simulink model "ssc_hydraulic_actuator_analog_control"  (R2020a)
settings: Solver=VariableStepAuto  StartTime=0.0  StopTime=10  MaxStep=0.02  RelTol=1e-3  AbsTol=1e-3  EnableMultiTasking=on
libraries: fl_lib x66, nesl_utility x3
CloseFcn:
  | try,close(h1_ssc_hydraulic_actuator_analog_control),end
  | clear h1_ssc_hydraulic_actuator_analog_control
  | 
  | clear simlog_ssc_hydraulic_actuator_analog_control
Description:
  | Hydraulic Actuator with Analog Position Controller
settings Model: Creator=MathWorks  LastModifiedBy=victo
settings SolverCC: AutoScaleAbsTol=off
settings DataIOCC: LimitDataPoints=on  SaveFormat=Array  ReturnWorkspaceOutputs=off
settings OptimizationCC: LifeSpan=inf
settings DebuggingCC: SolverPrmCheckMsg=warning  AllowSymbolicDim=off  PregeneratedLibrarySubsystemCodeDiagnostic=none  SFUnexpectedBacktrackingDiag=warning  SFNoUnconditionalDefaultTransitionDiag=warning  SFExecutionAtInitializationDiag=none  ArithmeticOperatorsInVariantConditions=warning
settings HardwareCC: ProdBitPerPointer=32  ProdBitPerSizeT=32  ProdBitPerPtrDiffT=32  ProdLargestAtomicFloat=None  ProdIntDivRoundTo=Undefined  ProdEndianess=Unspecified  ProdWordSize=32  ProdHWDeviceType=32-bit Generic
settings ModelReferenceCC: PropagateSignalLabelsOutOfModel=off
settings SFSimCC: SimUseLocalCustomCode=off  CustomCodeUndefinedFunction=UseInterfaceOnly
settings RTWCC: RTWUseLocalCustomCode=off
settings CodeAppCC: StateflowObjectComments=on
settings GRTTargetCC: TargetLangStandard=C89/C90 (ANSI)
settings ConfigComp: CovMetricSettings=dw  CovHtmlReporting=on  CovSaveCumulativeToWorkspaceVar=on  CovSaveSingleToWorkspaceVar=on  CovExternalEMLEnable=off  CovSFcnEnable=off
settings SimscapeCC: SimscapeLogType=all  SimscapeLogSimulationStatistics=on  SimscapeLogName=simlog_ssc_hydraulic_actuator_analog_control  SimscapeLogDataHistory=10000

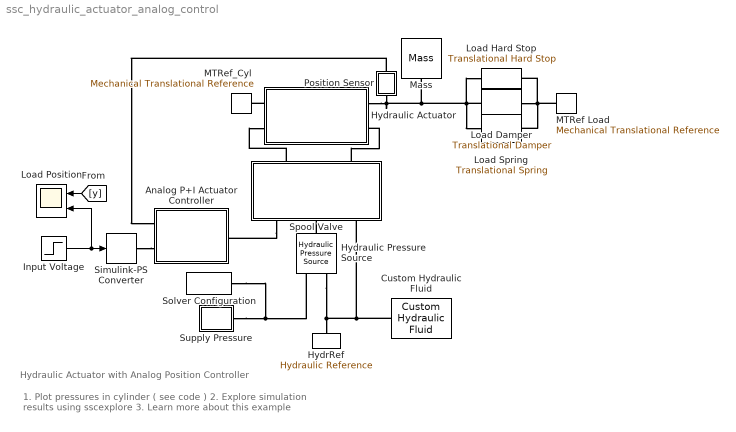
== system ssc_hydraulic_actuator_analog_control ==
  note: 1. Plot pressures in cylinder ( see code )
      | 2. Explore simulation results using sscexplore
      | 3. Learn more about this example
  note: Hydraulic Actuator with Analog Position Controller
  Analog P+I Actuator Controller : Subsystem
  Custom Hydraulic Fluid : fl_lib/Hydraulic/Hydraulic Utilities/Custom Hydraulic Fluid  density=850 kg/m^3  viscosity_kin=1.8e-05 m^2/s  bulk=8e+08 Pa  alpha=0.005  range_error=2
      settings: SourceProductName=Foundation Library  InternalSimscapePortConfiguration="{\"Bottom\":[],\"Left\":[],\"Right\":[{\"id\":\"G\",\"label\":\"\",\"type\":\"foundation.hydraulic.hydraulic\"}],\"Top\":[]}"
  HydrRef : fl_lib/Hydraulic/Hydraulic Elements/Hydraulic Reference
      settings: SourceProductName=Foundation Library
  Hydraulic Pressure Source : fl_lib/Hydraulic/Hydraulic Sources/Hydraulic Pressure Source
      settings: SourceProductName=Foundation Library  InternalSimscapePortConfiguration="{\"Bottom\":[],\"Left\":[{\"id\":\"P\",\"label\":\"P\",\"type\":\"foundation.hydraulic.hydraulic\"}],\"Right\":[{\"id\":\"S\",\"label\":\"S\",\"type\":\"input\"},{\"id\":\"T\",\"label\":\"T\",\"type\":\"foundation.hydraulic.hydraulic\"}],\"Top\":[]}"
  Hydraulic Actuator : Subsystem  mask(Double-Acting Hydraulic Actuator){A=5e-4, V=10e-6, PA=100, PB=100}
      mask prompts: A "Piston area (m^2)"; V "Chamber dead volume (m^3)"; PA "Positive-acting chamber A initial pressure (bar)"; PB "Negative-acting chamber B initial pressure (bar)"
      mask help: Models a double-acting hydraulic actuator using foundation library blocks
      mask Display:
      | plot([127.790967235342;156.136468285695;156.136468285695;127.790967235342;127.790967235342], [113.618216710165;113.618216710165;56.927214609459;56.927214609459;113.618216710165])
      | plot([261.014822172001;326.209474587813], [85.2727156598121;85.2727156598121])
      | plot([212.827470386401;212.827470386401;326.209474587813], [56.927214609459;28.581713559106;28.581713559106])
      | patch([0;326.445687096566;326.445687096566;0;0;0.472425017505884;0.472425017505884;325.97326207906;325.97326207906;0.472425017505884;0], [113.854429218918;113.854429218918;0;0;113.854429218918;113.382004201412;0.472425017505884;0.472425017505884;113.382004201412;113.382004201412;113.854429218918], [1;1;1])
      | plot([227.000220911577;227.000220911577;82.4381655547768;82.4381655547768;227.000220911577;227.000220911577], [99.4454661849886;113.618216710165;113.618216710165;56.927214609459;56.927214609459;71.0999651346356])
      | plot([82.4381655547768;54.0926645044237;82.4381655547768], [113.618216710165;85.2727156598121;56.927214609459])
      | plot([156.136468285695;261.014822172001;261.014822172001;156.136468285695;156.136468285695], [99.4454661849886;99.4454661849886;71.0999651346356;71.0999651346356;99.4454661849886])
      | plot([0.236212508752942;110.78366660513;110.78366660513], [28.581713559106;28.581713559106;56.927214609459])
      | plot([54.0926645044237;0.236212508752942], [85.2727156598121;85.2727156598121])
      | 
      | color('red');
      | port_label('LConn',1,'C');
      | port_label('LConn',2,'A');
      | port_label('RConn',1,'R');
      | port_label('RConn',2,'B');
      | color('black');
  Input Voltage : Step  Time=0.2  Before=2.5  After=3.0  SampleTime=0
  Load Position : Scope  NumInputPorts=2
  Load Damper : fl_lib/Mechanical/Translational Elements/Translational Damper  D=5000 N/(m/s)  v_specify=off  v_priority=High  v=0 m/s  v_nominal_specify=off  v_nominal_unit=m/s  v_nominal_value=1  f_specify=off  f_priority=High  f=0 N  f_nominal_specify=off  f_nominal_unit=N  f_nominal_value=1
      settings: SourceProductName=Foundation Library
  Load Hard Stop : fl_lib/Mechanical/Translational Elements/Translational Hard Stop  upper_bnd=50 mm  lower_bnd=-50 mm  stiff_up=1e+07 N/m  stiff_low=1e+07 N/m  D_up=3000 N/(m/s)  D_low=3000 N/(m/s)  model=3  transition=0.1 mm  v_specify=off  v_priority=High  v=0 m/s  v_nominal_specify=off  v_nominal_unit=m/s  v_nominal_value=1  f_specify=off  f_priority=High  f=0 N  f_nominal_specify=off  f_nominal_unit=N  f_nominal_value=1  x_specify=on  x_priority=High  x=0 m  x_nominal_specify=off  x_nominal_unit=m  x_nominal_value=1
      settings: SourceProductName=Foundation Library
  Load Spring : fl_lib/Mechanical/Translational Elements/Translational Spring  spr_rate=100000 N/m  v_specify=off  v_priority=High  v=0 m/s  v_nominal_specify=off  v_nominal_unit=m/s  v_nominal_value=1  f_specify=off  f_priority=High  f=0 N  f_nominal_specify=off  f_nominal_unit=N  f_nominal_value=1  x_specify=off  x_priority=High  x=0 mm  x_nominal_specify=off  x_nominal_unit=m  x_nominal_value=1
      settings: SourceProductName=Foundation Library
  MTRef Load : fl_lib/Mechanical/Translational Elements/Mechanical Translational Reference
      settings: SourceProductName=Foundation Library
  MTRef_Cyl : fl_lib/Mechanical/Translational Elements/Mechanical Translational Reference
      settings: SourceProductName=Foundation Library
  Mass : fl_lib/Mechanical/Translational Elements/Mass  mass=20 kg  v_specify=off  v_priority=High  v=0 m/s  v_nominal_specify=off  v_nominal_unit=m/s  v_nominal_value=1  f_specify=off  f_priority=High  f=0 N  f_nominal_specify=off  f_nominal_unit=N  f_nominal_value=1
      settings: SourceProductName=Foundation Library
  Position Sensor : Subsystem
      mask Display: disp('y')
  Simulink-PS Converter : nesl_utility/Simulink-PS Converter  PhysicalDomain=network_engine_domain  SubClassName=ps_input  LeftPortType=input  RightPortType=output  PseudoPeriodic=off  Frequencies=[]  NoiseDistribution=none  NoiseParameters=[]  Unit=V  AffineConversion=off  FilteringAndDerivatives=zero  SimscapeFilterOrder=1  InputFilterTimeConstant=.001  UdotUserProvided=0
      settings: SourceProductName=Utilities
  Solver Configuration : nesl_utility/Solver Configuration  PhysicalDomain=network_engine_domain  SubClassName=solver  LeftPortType=input  RightPortType=generic  Tones=[]  Harmonics=[]  SimulateNoise=off  Profile=off  UseLocalSampling=off  EnableSwitchedLinearOptims=on  FrequencyDomain=off  UseCCode=off  RelTol=0.001  AbsTol=1e-06  MinStep=1e-09  ToWorkspace=off  RevertToSquareIcSolve=off  NumHomotopyIterations=100  PhasorMode=off  PhasorModeNumHarmonics=1  DoDC=off  ResidualTolerance=1e-9  UseLocalSolver=off  LocalSolverChoice=NE_BACKWARD_EULER_ADVANCER  LocalSolverSampleTime=0.001  DoFixedCost=off  MaxNonlinIter=3  MaxModeIter=2  LinearAlgebra=auto  EquationFormulation=NE_TIME_EF  DelaysMemoryBudget=1024  AutomaticFiltering=on  FilteringTimeConstant=0.001  PartitionStorageMethod=AS_NEEDED  PartitionMemoryBudget=1024  PartitionMethod=ROBUST
      settings: SourceProductName=Utilities
  Spool Valve : Subsystem  Tag=PublishSubsystem  mask(Single-Stage Servo Valve){K_V=0.5, x_max=0.5, A_max=9, x_lap=0.02, A_leak=0.25, G=0.5e-3/(pi/2), J=1e-4, lambda=0.01, R=10, L=2.5, Kt=0.04, R_controller=[10e3 10e3 10e3 100e3 50 100e3 10e3]}
      mask prompts: K_V "Flow Coefficient:"; x_max "Spool displacement limit (mm)"; A_max "Maximum orifice area (mm^2)"; x_lap "Spool displacement range for leakage (mm)"; A_leak "Leakage area at x=0 (mm^2)"; G "Spool displacement per motor rotation (m/radian)"; J "Total inertia reflected to motor (kg m^2)"; lambda "Total damping reflected to motor (Nm/(rad/s))"; R "Torque motor winding resistance (ohms)"; L "Torque motor winding inductance (H)"; Kt "Torque motor torque constant (Nm/A)"; R_controller "Motor controller resistance values [R1 R2 R3 R4 R5 R6 R7] (ohms)"
      mask help: Models a spool valve actuated directly by a torque motor.
      mask Display:
      | % Plot icon
      | plot([0;337.311462499201;337.311462499201;0;0], [566.910021007061;566.910021007061;0;0;566.910021007061])
      | plot([84.6585631370544;241.503668949008], [353;353])
      | plot([84.6585631370544;241.503668949008], [214;214])
      | plot([84.6585631370544;241.503668949008;241.503668949008;84.6585631370544;84.6585631370544], [491;491;76;76;491])
      | plot([84.6585631370544;241.503668949008], [449;449])
      | plot([241.503668949008;210.071657784283], [310;310])
      | plot([210.071657784283;210.071657784283;210.071657784283], [326;295;310.414731502533])
      | plot([241.503668949008;210.071657784283], [257;257])
      | plot([210.071657784283;210.071657784283;210.071657784283], [272;241;236.464468762279])
      | plot([84.6585631370544;115.964594297111], [257;257])
      | plot([115.964594297111;115.964594297111;115.964594297111], [272;241;236.464468762279])
      | plot([84.6585631370544;115.964594297111], [310;310])
      | plot([115.964594297111;115.964594297111;115.964594297111], [326;295;310.414731502533])
      | plot([84.6585631370544;241.503668949008], [185;110])
      | plot([241.503668949008;84.6585631370544], [185;110])
      | plot([84.6585631370544;241.503668949008], [395;395])
      | patch([85.0365031510592;110.547454096377;121.885654516518;85.0365031510592], [110;140;120;110], [0;0;0])
      | plot([85.0365031510592;110.547454096377;121.885654516518;85.0365031510592], [110;140;120;110])
      | patch([240.936758928001;204.087607562542;215.425807982683;240.936758928001], [109;120;140;109], [0;0;0])
      | 
      | plot([240.936758928001;204.087607562542;215.425807982683;240.936758928001], [109;120;140;109])
      | patch([83.6507230997086;127.554754726589;127.554754726589;83.6507230997086], [394;405;384;394], [0;0;0])
      | plot([83.6507230997086;127.554754726589;127.554754726589;83.6507230997086], [394;405;384;394])
      | patch([245.283069089055;201.253057457507;201.253057457507;245.283069089055], [451;461;440;451], [0;0;0])
      | plot([245.283069089055;201.253057457507;201.253057457507;245.283069089055], [451;461;440;451])
      | 
      | % Port labels
      | color('red')
      | port_label('LConn', 1,'S')
      | port_label('LConn', 2,'P')
      | port_label('LConn', 3,'T')
      | port_label('RConn', 1,'A')
      | port_label('RConn', 2,'B')
      | color('black')
  Supply Pressure : Subsystem
  wires:
  Input Voltage/1 -> Load Position/2, Simulink-PS Converter/1
  [y] -> Load Position/1
  connections:
  Spool Valve/LConn1 -- Analog P+I Actuator Controller/RConn1
  Custom Hydraulic Fluid/RConn1 -- Hydraulic Pressure Source/RConn2 -- HydrRef/LConn1 -- Spool Valve/LConn3
  Spool Valve/RConn2 -- Hydraulic Actuator/RConn2
  Spool Valve/RConn1 -- Hydraulic Actuator/LConn2
  Simulink-PS Converter/RConn1 -- Analog P+I Actuator Controller/LConn2
  Hydraulic Pressure Source/LConn1 -- Spool Valve/LConn2
  Load Spring/LConn1 -- Load Damper/LConn1 -- Mass/LConn1 -- Position Sensor/RConn1 -- Hydraulic Actuator/RConn1 -- Load Hard Stop/LConn1
  Position Sensor/LConn1 -- Analog P+I Actuator Controller/LConn1
  Hydraulic Actuator/LConn1 -- MTRef_Cyl/LConn1
  Supply Pressure/RConn1 -- Solver Configuration/RConn1 -- Hydraulic Pressure Source/RConn1
  Load Hard Stop/RConn1 -- Load Damper/RConn1 -- MTRef Load/LConn1 -- Load Spring/RConn1

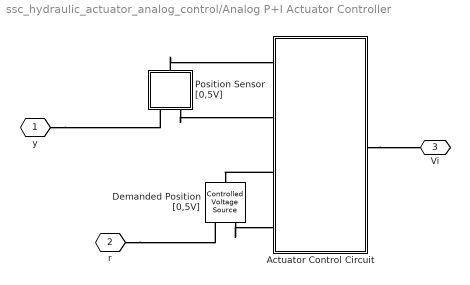
== system ssc_hydraulic_actuator_analog_control/Analog P+I Actuator Controller ==
  Actuator Control Circuit : Subsystem  Tag=PublishSubsystem
  Demanded Position [0,5V] : fl_lib/Electrical/Electrical Sources/Controlled Voltage Source
      settings: SourceProductName=Foundation Library
  Position Sensor [0,5V] : Subsystem
  y : PMIOPort  Tag=PMCPort  Side=Left
  r : PMIOPort  Tag=PMCPort  Port=2  Side=Left
  Vi : PMIOPort  Port=3  Side=Right
  connections:
  y/RConn1 -- Position Sensor [0,5V]/LConn1
  r/RConn1 -- Demanded Position [0,5V]/RConn1
  Actuator Control Circuit/LConn3 -- Demanded Position [0,5V]/LConn1
  Position Sensor [0,5V]/RConn1 -- Actuator Control Circuit/LConn1
  Position Sensor [0,5V]/LConn2 -- Actuator Control Circuit/LConn2
  Actuator Control Circuit/RConn1 -- Vi/RConn1
  Demanded Position [0,5V]/RConn2 -- Actuator Control Circuit/LConn4

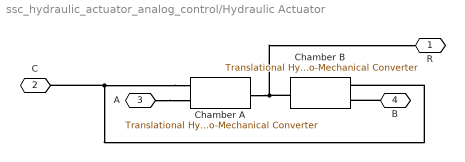
== system ssc_hydraulic_actuator_analog_control/Hydraulic Actuator ==
  Chamber A : fl_lib/Hydraulic/Hydraulic Elements/Translational Hydro-Mechanical Converter  area=A m^2  or=1  compressibility=1  init_pos=0 m  V_dead=V m^3  k_sh=1.4  initial_pressure=PA bar
      settings: SourceProductName=Foundation Library  InternalSimscapePortConfiguration="{\"Bottom\":[],\"Left\":[{\"id\":\"C\",\"label\":\"C\",\"type\":\"foundation.mechanical.translational.translational\"},{\"id\":\"A\",\"label\":\"A\",\"type\":\"foundation.hydraulic.hydraulic\"}],\"Right\":[{\"id\":\"R\",\"label\":\"R\",\"type\":\"foundation.mechanical.translational.translational\"}],\"Top\":[]}"
  Chamber B : fl_lib/Hydraulic/Hydraulic Elements/Translational Hydro-Mechanical Converter  area=A m^2  or=2  compressibility=1  init_pos=50 mm  V_dead=V m^3  k_sh=1.4  initial_pressure=PB bar
      settings: SourceProductName=Foundation Library  InternalSimscapePortConfiguration="{\"Bottom\":[],\"Left\":[{\"id\":\"C\",\"label\":\"C\",\"type\":\"foundation.mechanical.translational.translational\"},{\"id\":\"A\",\"label\":\"A\",\"type\":\"foundation.hydraulic.hydraulic\"}],\"Right\":[{\"id\":\"R\",\"label\":\"R\",\"type\":\"foundation.mechanical.translational.translational\"}],\"Top\":[]}"
  R : PMIOPort  Side=Right
  C : PMIOPort  Port=2  Side=Left
  A : PMIOPort  Port=3  Side=Left
  B : PMIOPort  Port=4  Side=Right
  connections:
  B/RConn1 -- Chamber B/LConn2
  Chamber A/RConn1 -- Chamber B/RConn1 -- R/RConn1
  A/RConn1 -- Chamber A/LConn2
  Chamber A/LConn1 -- C/RConn1 -- Chamber B/LConn1

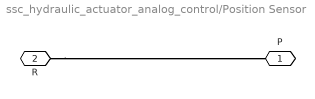
== system ssc_hydraulic_actuator_analog_control/Position Sensor ==
  P : PMIOPort  Side=Left
  R : PMIOPort  Port=2  Side=Right
  connections:
  R/RConn1 -- P/RConn1

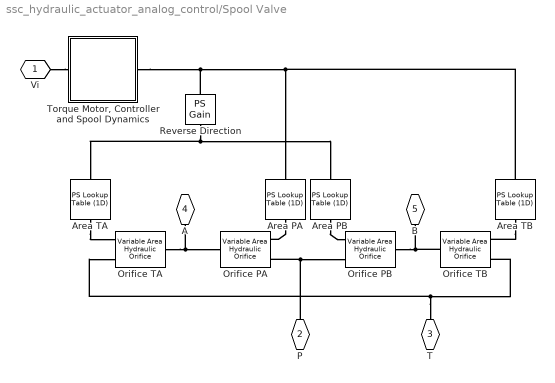
== system ssc_hydraulic_actuator_analog_control/Spool Valve ==
  Area PA : fl_lib/Physical Signals/Lookup Tables/PS Lookup Table (1D)  x=[-x_max -x_lap 0 x_lap x_max 2*x_max] mm  f=[0 0 A_leak 2*A_leak A_max A_max] mm^2  interp_method=simscape.enum.interpolation.linear  extrap_method=simscape.enum.extrapolation.linear
      settings: SourceProductName=Foundation Library
  Area PB : fl_lib/Physical Signals/Lookup Tables/PS Lookup Table (1D)  x=[-x_max -x_lap 0 x_lap x_max 2*x_max] mm  f=[0 0 A_leak 2*A_leak A_max A_max] mm^2  interp_method=simscape.enum.interpolation.linear  extrap_method=simscape.enum.extrapolation.linear
      settings: SourceProductName=Foundation Library
  Area TA : fl_lib/Physical Signals/Lookup Tables/PS Lookup Table (1D)  x=[-x_max -x_lap 0 x_lap x_max 2*x_max] mm  f=[0 0 A_leak 2*A_leak A_max A_max] mm^2  interp_method=simscape.enum.interpolation.linear  extrap_method=simscape.enum.extrapolation.linear
      settings: SourceProductName=Foundation Library
  Area TB : fl_lib/Physical Signals/Lookup Tables/PS Lookup Table (1D)  x=[-x_max -x_lap 0 x_lap x_max 2*x_max] mm  f=[0 0 A_leak 2*A_leak A_max A_max] mm^2  interp_method=simscape.enum.interpolation.linear  extrap_method=simscape.enum.extrapolation.linear
      settings: SourceProductName=Foundation Library
  Orifice PA : fl_lib/Hydraulic/Hydraulic Elements/Variable Area Hydraulic Orifice  C_d=K_V  min_area=1e-12 m^2  lam_spec=1  B_lam=0.999  Re_cr=12  q_specify=off  q_priority=High  q=1 m^3/s  q_nominal_specify=off  q_nominal_unit=m^3/s  q_nominal_value=1  p_specify=off  p_priority=High  p=0 Pa  p_nominal_specify=off  p_nominal_unit=Pa  p_nominal_value=1
      settings: SourceProductName=Foundation Library  InternalSimscapePortConfiguration="{\"Bottom\":[],\"Left\":[{\"id\":\"AR\",\"label\":\"AR\",\"type\":\"input\"},{\"id\":\"A\",\"label\":\"A\",\"type\":\"foundation.hydraulic.hydraulic\"}],\"Right\":[{\"id\":\"B\",\"label\":\"B\",\"type\":\"foundation.hydraulic.hydraulic\"}],\"Top\":[]}"
  Orifice PB : fl_lib/Hydraulic/Hydraulic Elements/Variable Area Hydraulic Orifice  C_d=K_V  min_area=1e-12 m^2  lam_spec=1  B_lam=0.999  Re_cr=12  q_specify=off  q_priority=High  q=1 m^3/s  q_nominal_specify=off  q_nominal_unit=m^3/s  q_nominal_value=1  p_specify=off  p_priority=High  p=0 Pa  p_nominal_specify=off  p_nominal_unit=Pa  p_nominal_value=1
      settings: SourceProductName=Foundation Library  InternalSimscapePortConfiguration="{\"Bottom\":[],\"Left\":[{\"id\":\"AR\",\"label\":\"AR\",\"type\":\"input\"},{\"id\":\"A\",\"label\":\"A\",\"type\":\"foundation.hydraulic.hydraulic\"}],\"Right\":[{\"id\":\"B\",\"label\":\"B\",\"type\":\"foundation.hydraulic.hydraulic\"}],\"Top\":[]}"
  Orifice TA : fl_lib/Hydraulic/Hydraulic Elements/Variable Area Hydraulic Orifice  C_d=K_V  min_area=1e-12 m^2  lam_spec=1  B_lam=0.999  Re_cr=12  q_specify=off  q_priority=High  q=1 m^3/s  q_nominal_specify=off  q_nominal_unit=m^3/s  q_nominal_value=1  p_specify=off  p_priority=High  p=0 Pa  p_nominal_specify=off  p_nominal_unit=Pa  p_nominal_value=1
      settings: SourceProductName=Foundation Library  InternalSimscapePortConfiguration="{\"Bottom\":[],\"Left\":[{\"id\":\"AR\",\"label\":\"AR\",\"type\":\"input\"},{\"id\":\"A\",\"label\":\"A\",\"type\":\"foundation.hydraulic.hydraulic\"}],\"Right\":[{\"id\":\"B\",\"label\":\"B\",\"type\":\"foundation.hydraulic.hydraulic\"}],\"Top\":[]}"
  Orifice TB : fl_lib/Hydraulic/Hydraulic Elements/Variable Area Hydraulic Orifice  C_d=K_V  min_area=1e-12 m^2  lam_spec=1  B_lam=0.999  Re_cr=12  q_specify=off  q_priority=High  q=1 m^3/s  q_nominal_specify=off  q_nominal_unit=m^3/s  q_nominal_value=1  p_specify=off  p_priority=High  p=0 Pa  p_nominal_specify=off  p_nominal_unit=Pa  p_nominal_value=1
      settings: SourceProductName=Foundation Library  InternalSimscapePortConfiguration="{\"Bottom\":[],\"Left\":[{\"id\":\"AR\",\"label\":\"AR\",\"type\":\"input\"},{\"id\":\"A\",\"label\":\"A\",\"type\":\"foundation.hydraulic.hydraulic\"}],\"Right\":[{\"id\":\"B\",\"label\":\"B\",\"type\":\"foundation.hydraulic.hydraulic\"}],\"Top\":[]}"
  Reverse Direction : fl_lib/Physical Signals/Functions/PS Gain  gain=-1
      settings: SourceProductName=Foundation Library
  "Torque Motor, Controller and Spool Dynamics" : Subsystem
  Vi : PMIOPort  Tag=PMCPort  Side=Left
  P : PMIOPort  Tag=PMCPort  Port=2  Side=Left
  T : PMIOPort  Tag=PMCPort  Port=3  Side=Left
  A : PMIOPort  Tag=PMCPort  Port=4  Side=Right
  B : PMIOPort  Tag=PMCPort  Port=5  Side=Right
  connections:
  B/RConn1 -- Orifice PB/RConn1 -- Orifice TB/RConn1
  T/RConn1 -- Orifice TA/LConn2 -- Orifice TB/LConn2
  A/RConn1 -- Orifice PA/RConn1 -- Orifice TA/RConn1
  P/RConn1 -- Orifice PB/LConn2 -- Orifice PA/LConn2
  Vi/RConn1 -- "Torque Motor, Controller and Spool Dynamics"/LConn1
  Reverse Direction/RConn1 -- Area PB/LConn1 -- Area TA/LConn1
  Area TB/RConn1 -- Orifice TB/LConn1
  Area PA/RConn1 -- Orifice PA/LConn1
  "Torque Motor, Controller and Spool Dynamics"/RConn1 -- Area TB/LConn1 -- Area PA/LConn1 -- Reverse Direction/LConn1
  Area TA/RConn1 -- Orifice TA/LConn1
  Area PB/RConn1 -- Orifice PB/LConn1

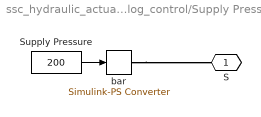
== system ssc_hydraulic_actuator_analog_control/Supply Pressure ==
  Supply Pressure : Constant  Value=200
  bar : nesl_utility/Simulink-PS Converter  PhysicalDomain=network_engine_domain  SubClassName=ps_input  LeftPortType=input  RightPortType=output  PseudoPeriodic=off  Frequencies=[]  NoiseDistribution=none  NoiseParameters=[]  Unit=bar  AffineConversion=off  FilteringAndDerivatives=zero  SimscapeFilterOrder=1  InputFilterTimeConstant=.001  UdotUserProvided=0
      settings: SourceProductName=Utilities
  S : PMIOPort  Side=Right
  wires:
  Supply Pressure/1 -> bar/1
  connections:
  bar/RConn1 -- S/RConn1

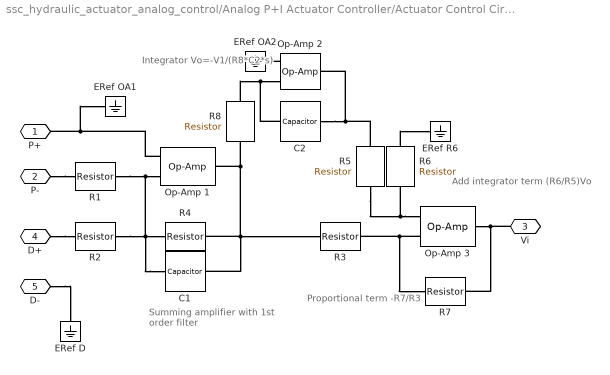
== system ssc_hydraulic_actuator_analog_control/Analog P+I Actuator Controller/Actuator Control Circuit ==
  note: Summing amplifier
      | with 1st order filter
  note: Integrator
      | Vo=-V1/(R8*C2*s)
  note: Proportional
      | term -R7/R3
  note: Add integrator
      | term (R6/R5)Vo
  C1 : fl_lib/Electrical/Electrical Elements/Capacitor  c=0.15e-06 F  r=1e-06 Ohm  g=0 1/Ohm  i_specify=off  i_priority=High  i=0 A  i_nominal_specify=off  i_nominal_unit=A  i_nominal_value=1  v_specify=off  v_priority=High  v=0 V  v_nominal_specify=off  v_nominal_unit=V  v_nominal_value=1  vc_specify=on  vc_priority=High  vc=0 V  vc_nominal_specify=off  vc_nominal_unit=V  vc_nominal_value=1
      settings: SourceProductName=Foundation Library
  C2 : fl_lib/Electrical/Electrical Elements/Capacitor  c=100e-06 F  r=1e-06 Ohm  g=0 1/Ohm  i_specify=off  i_priority=High  i=0 A  i_nominal_specify=off  i_nominal_unit=A  i_nominal_value=1  v_specify=off  v_priority=High  v=0 V  v_nominal_specify=off  v_nominal_unit=V  v_nominal_value=1  vc_specify=on  vc_priority=High  vc=0 V  vc_nominal_specify=off  vc_nominal_unit=V  vc_nominal_value=1
      settings: SourceProductName=Foundation Library
  ERef D : fl_lib/Electrical/Electrical Elements/Electrical Reference
      settings: SourceProductName=Foundation Library
  ERef OA1 : fl_lib/Electrical/Electrical Elements/Electrical Reference
      settings: SourceProductName=Foundation Library
  ERef OA2 : fl_lib/Electrical/Electrical Elements/Electrical Reference
      settings: SourceProductName=Foundation Library
  ERef R6 : fl_lib/Electrical/Electrical Elements/Electrical Reference
      settings: SourceProductName=Foundation Library
  Op-Amp 1 : fl_lib/Electrical/Electrical Elements/Op-Amp  outI_specify=off  outI_priority=High  outI=0 A  outI_nominal_specify=off  outI_nominal_unit=A  outI_nominal_value=1
      settings: SourceProductName=Foundation Library
  Op-Amp 2 : fl_lib/Electrical/Electrical Elements/Op-Amp  outI_specify=off  outI_priority=High  outI=0 A  outI_nominal_specify=off  outI_nominal_unit=A  outI_nominal_value=1
      settings: SourceProductName=Foundation Library
  Op-Amp 3 : fl_lib/Electrical/Electrical Elements/Op-Amp  outI_specify=off  outI_priority=High  outI=0 A  outI_nominal_specify=off  outI_nominal_unit=A  outI_nominal_value=1
      settings: SourceProductName=Foundation Library
  R{1..3,5..6,8} (6 alike) : fl_lib/Electrical/Electrical Elements/Resistor  R=10e3 Ohm  i_specify=off  i_priority=High  i=0 A  i_nominal_specify=off  i_nominal_unit=A  i_nominal_value=1  v_specify=off  v_priority=High  v=0 V  v_nominal_specify=off  v_nominal_unit=V  v_nominal_value=1
      settings: SourceProductName=Foundation Library
  R4 : fl_lib/Electrical/Electrical Elements/Resistor  R=5.7e3 Ohm  i_specify=off  i_priority=High  i=0 A  i_nominal_specify=off  i_nominal_unit=A  i_nominal_value=1  v_specify=off  v_priority=High  v=0 V  v_nominal_specify=off  v_nominal_unit=V  v_nominal_value=1
      settings: SourceProductName=Foundation Library
  R7 : fl_lib/Electrical/Electrical Elements/Resistor  R=20e3 Ohm  i_specify=off  i_priority=High  i=0 A  i_nominal_specify=off  i_nominal_unit=A  i_nominal_value=1  v_specify=off  v_priority=High  v=0 V  v_nominal_specify=off  v_nominal_unit=V  v_nominal_value=1
      settings: SourceProductName=Foundation Library
  P+ : PMIOPort  Side=Left
  P- : PMIOPort  Port=2  Side=Left
  Vi : PMIOPort  Port=3  Side=Right
  D+ : PMIOPort  Port=4  Side=Left
  D- : PMIOPort  Port=5  Side=Left
  connections:
  C1/LConn1 -- R2/RConn1 -- R1/RConn1 -- Op-Amp 1/LConn2 -- R4/LConn1
  R4/RConn1 -- C1/RConn1 -- R3/LConn1 -- Op-Amp 1/RConn1 -- R8/LConn1
  C2/LConn1 -- Op-Amp 2/LConn2 -- R8/RConn1
  C2/RConn1 -- R5/LConn1 -- Op-Amp 2/RConn1
  Op-Amp 1/LConn1 -- P+/RConn1 -- ERef OA1/LConn1
  R6/RConn1 -- ERef R6/LConn1
  Op-Amp 2/LConn1 -- ERef OA2/LConn1
  Op-Amp 3/RConn1 -- Vi/RConn1 -- R7/RConn1
  Op-Amp 3/LConn1 -- R5/RConn1 -- R6/LConn1
  Op-Amp 3/LConn2 -- R3/RConn1 -- R7/LConn1
  P-/RConn1 -- R1/LConn1
  D+/RConn1 -- R2/LConn1
  D-/RConn1 -- ERef D/LConn1

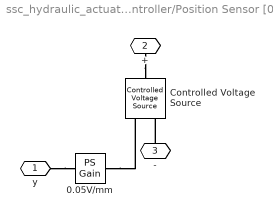
== system ssc_hydraulic_actuator_analog_control/Analog P+I Actuator Controller/Position Sensor [0,5V] ==
  0.05V/mm : fl_lib/Physical Signals/Functions/PS Gain  gain=5/100 V/mm
      settings: SourceProductName=Foundation Library
  Controlled Voltage Source : fl_lib/Electrical/Electrical Sources/Controlled Voltage Source
      settings: SourceProductName=Foundation Library
  y : PMIOPort  Side=Left
  + : PMIOPort  Port=2  Side=Right
  - : PMIOPort  Port=3  Side=Left
  connections:
  0.05V/mm/RConn1 -- Controlled Voltage Source/RConn1
  +/RConn1 -- Controlled Voltage Source/LConn1
  -/RConn1 -- Controlled Voltage Source/RConn2
  y/RConn1 -- 0.05V/mm/LConn1

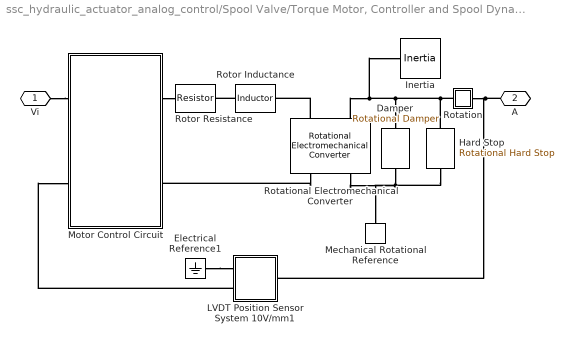
== system ssc_hydraulic_actuator_analog_control/Spool Valve/Torque Motor, Controller and Spool Dynamics ==
  Damper : fl_lib/Mechanical/Rotational Elements/Rotational Damper  D=lambda N*m/(rad/s)  w_specify=off  w_priority=High  w=0 rad/s  w_nominal_specify=off  w_nominal_unit=rad/s  w_nominal_value=1  t_specify=off  t_priority=High  t=0 N*m  t_nominal_specify=off  t_nominal_unit=N*m  t_nominal_value=1
      settings: SourceProductName=Foundation Library
  Electrical Reference1 : fl_lib/Electrical/Electrical Elements/Electrical Reference
      settings: SourceProductName=Foundation Library
  Hard Stop : fl_lib/Mechanical/Rotational Elements/Rotational Hard Stop  upper_bnd=x_max*1e-3/G rad  lower_bnd=-x_max*1e-3/G rad  stiff_up=1e+06 N*m/rad  stiff_low=1e+6 N*m/rad  D_up=0.05 N*m/(rad/s)  D_low=0.05 N*m/(rad/s)  model=3  transition=0.001 rad  w_specify=off  w_priority=High  w=0 rad/s  w_nominal_specify=off  w_nominal_unit=rad/s  w_nominal_value=1  t_specify=off  t_priority=High  t=0 N*m  t_nominal_specify=off  t_nominal_unit=N*m  t_nominal_value=1  phi_specify=on  phi_priority=High  phi=0 rad  phi_nominal_specify=off  phi_nominal_unit=rad  phi_nominal_value=1
      settings: SourceProductName=Foundation Library
  Inertia : fl_lib/Mechanical/Rotational Elements/Inertia  inertia=J kg*m^2  w_specify=off  w_priority=High  w=0 rad/s  w_nominal_specify=off  w_nominal_unit=rad/s  w_nominal_value=1  t_specify=off  t_priority=High  t=0 N*m  t_nominal_specify=off  t_nominal_unit=N*m  t_nominal_value=1
      settings: SourceProductName=Foundation Library
  LVDT Position Sensor System 10V/mm1 : Subsystem
  Mechanical Rotational Reference : fl_lib/Mechanical/Rotational Elements/Mechanical Rotational Reference
      settings: SourceProductName=Foundation Library
  Motor Control Circuit : Subsystem  Tag=PublishSubsystem
  Rotation : Subsystem
      mask Display: disp('A')
  Rotational Electromechanical Converter : fl_lib/Electrical/Electrical Elements/Rotational Electromechanical Converter  K=Kt V/(rad/s)  i_specify=off  i_priority=High  i=0 A  i_nominal_specify=off  i_nominal_unit=A  i_nominal_value=1  v_specify=off  v_priority=High  v=0 V  v_nominal_specify=off  v_nominal_unit=V  v_nominal_value=1  t_specify=off  t_priority=High  t=0 N*m  t_nominal_specify=off  t_nominal_unit=N*m  t_nominal_value=1  w_specify=off  w_priority=High  w=0 rad/s  w_nominal_specify=off  w_nominal_unit=rad/s  w_nominal_value=1
      settings: SourceProductName=Foundation Library
  Rotor Inductance : fl_lib/Electrical/Electrical Elements/Inductor  l=L H  r=0 Ohm  g=1e-09 1/Ohm  i_specify=off  i_priority=High  i=0 A  i_nominal_specify=off  i_nominal_unit=A  i_nominal_value=1  v_specify=off  v_priority=High  v=0 V  v_nominal_specify=off  v_nominal_unit=V  v_nominal_value=1  i_L_specify=on  i_L_priority=High  i_L=0 A  i_L_nominal_specify=off  i_L_nominal_unit=A  i_L_nominal_value=1
      settings: SourceProductName=Foundation Library
  Rotor Resistance : fl_lib/Electrical/Electrical Elements/Resistor  Tag=Factory Generic  R=R Ohm  i_specify=off  i_priority=High  i=0 A  i_nominal_specify=off  i_nominal_unit=A  i_nominal_value=1  v_specify=off  v_priority=High  v=0 V  v_nominal_specify=off  v_nominal_unit=V  v_nominal_value=1
      settings: SourceProductName=Foundation Library
  Vi : PMIOPort  Side=Left
  A : PMIOPort  Port=2  Side=Right
  connections:
  Damper/RConn1 -- Hard Stop/RConn1 -- Rotational Electromechanical Converter/RConn2 -- Mechanical Rotational Reference/LConn1
  Rotational Electromechanical Converter/LConn1 -- Rotor Inductance/RConn1
  Rotor Inductance/LConn1 -- Rotor Resistance/RConn1
  Motor Control Circuit/RConn1 -- Rotor Resistance/LConn1
  Vi/RConn1 -- Motor Control Circuit/LConn1
  LVDT Position Sensor System 10V/mm1/RConn2 -- Motor Control Circuit/LConn2
  Rotational Electromechanical Converter/RConn1 -- Motor Control Circuit/RConn2
  Electrical Reference1/LConn1 -- LVDT Position Sensor System 10V/mm1/RConn1
  A/RConn1 -- Rotation/RConn1 -- LVDT Position Sensor System 10V/mm1/LConn1
  Hard Stop/LConn1 -- Rotation/LConn1 -- Rotational Electromechanical Converter/LConn2 -- Inertia/LConn1 -- Damper/LConn1

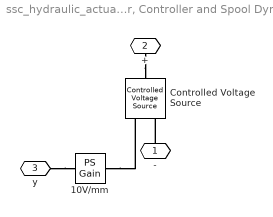
== system ssc_hydraulic_actuator_analog_control/Spool Valve/Torque Motor, Controller and Spool Dynamics/LVDT Position Sensor System 10V//mm1 ==
  10V/mm : fl_lib/Physical Signals/Functions/PS Gain  gain=10 V/mm
      settings: SourceProductName=Foundation Library
  Controlled Voltage Source : fl_lib/Electrical/Electrical Sources/Controlled Voltage Source
      settings: SourceProductName=Foundation Library
  - : PMIOPort  Side=Right
  + : PMIOPort  Port=2  Side=Right
  y : PMIOPort  Port=3  Side=Left
  connections:
  y/RConn1 -- 10V/mm/LConn1
  -/RConn1 -- Controlled Voltage Source/RConn2
  +/RConn1 -- Controlled Voltage Source/LConn1
  10V/mm/RConn1 -- Controlled Voltage Source/RConn1

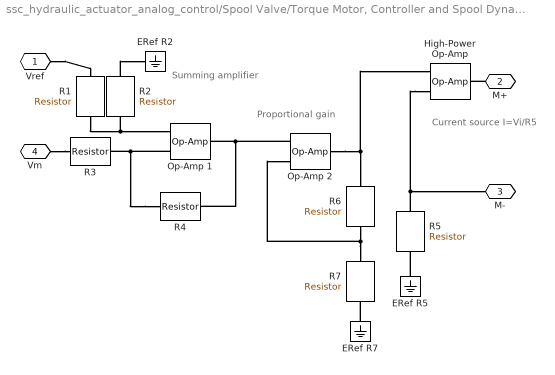
== system ssc_hydraulic_actuator_analog_control/Spool Valve/Torque Motor, Controller and Spool Dynamics/Motor Control Circuit ==
  note: Current source
      | I=Vi/R5
  note: Summing
      | amplifier
  note: Proportional gain
  ERef R2 : fl_lib/Electrical/Electrical Elements/Electrical Reference
      settings: SourceProductName=Foundation Library
  ERef R5 : fl_lib/Electrical/Electrical Elements/Electrical Reference
      settings: SourceProductName=Foundation Library
  ERef R7 : fl_lib/Electrical/Electrical Elements/Electrical Reference
      settings: SourceProductName=Foundation Library
  High-Power Op-Amp : fl_lib/Electrical/Electrical Elements/Op-Amp  outI_specify=off  outI_priority=High  outI=0 A  outI_nominal_specify=off  outI_nominal_unit=A  outI_nominal_value=1
      settings: SourceProductName=Foundation Library
  Op-Amp 1 : fl_lib/Electrical/Electrical Elements/Op-Amp  outI_specify=off  outI_priority=High  outI=0 A  outI_nominal_specify=off  outI_nominal_unit=A  outI_nominal_value=1
      settings: SourceProductName=Foundation Library
  Op-Amp 2 : fl_lib/Electrical/Electrical Elements/Op-Amp  outI_specify=off  outI_priority=High  outI=0 A  outI_nominal_specify=off  outI_nominal_unit=A  outI_nominal_value=1
      settings: SourceProductName=Foundation Library
  R1 : fl_lib/Electrical/Electrical Elements/Resistor  R=R_controller(1) Ohm  i_specify=off  i_priority=High  i=0 A  i_nominal_specify=off  i_nominal_unit=A  i_nominal_value=1  v_specify=off  v_priority=High  v=0 V  v_nominal_specify=off  v_nominal_unit=V  v_nominal_value=1
      settings: SourceProductName=Foundation Library
  R2 : fl_lib/Electrical/Electrical Elements/Resistor  R=R_controller(2) Ohm  i_specify=off  i_priority=High  i=0 A  i_nominal_specify=off  i_nominal_unit=A  i_nominal_value=1  v_specify=off  v_priority=High  v=0 V  v_nominal_specify=off  v_nominal_unit=V  v_nominal_value=1
      settings: SourceProductName=Foundation Library
  R3 : fl_lib/Electrical/Electrical Elements/Resistor  R=R_controller(3) Ohm  i_specify=off  i_priority=High  i=0 A  i_nominal_specify=off  i_nominal_unit=A  i_nominal_value=1  v_specify=off  v_priority=High  v=0 V  v_nominal_specify=off  v_nominal_unit=V  v_nominal_value=1
      settings: SourceProductName=Foundation Library
  R4 : fl_lib/Electrical/Electrical Elements/Resistor  R=R_controller(4) Ohm  i_specify=off  i_priority=High  i=0 A  i_nominal_specify=off  i_nominal_unit=A  i_nominal_value=1  v_specify=off  v_priority=High  v=0 V  v_nominal_specify=off  v_nominal_unit=V  v_nominal_value=1
      settings: SourceProductName=Foundation Library
  R5 : fl_lib/Electrical/Electrical Elements/Resistor  R=R_controller(5) Ohm  i_specify=off  i_priority=High  i=0 A  i_nominal_specify=off  i_nominal_unit=A  i_nominal_value=1  v_specify=off  v_priority=High  v=0 V  v_nominal_specify=off  v_nominal_unit=V  v_nominal_value=1
      settings: SourceProductName=Foundation Library
  R6 : fl_lib/Electrical/Electrical Elements/Resistor  R=R_controller(6) Ohm  i_specify=off  i_priority=High  i=0 A  i_nominal_specify=off  i_nominal_unit=A  i_nominal_value=1  v_specify=off  v_priority=High  v=0 V  v_nominal_specify=off  v_nominal_unit=V  v_nominal_value=1
      settings: SourceProductName=Foundation Library
  R7 : fl_lib/Electrical/Electrical Elements/Resistor  R=R_controller(7) Ohm  i_specify=off  i_priority=High  i=0 A  i_nominal_specify=off  i_nominal_unit=A  i_nominal_value=1  v_specify=off  v_priority=High  v=0 V  v_nominal_specify=off  v_nominal_unit=V  v_nominal_value=1
      settings: SourceProductName=Foundation Library
  Vref : PMIOPort  Side=Left
  M+ : PMIOPort  Port=2  Side=Right
  M- : PMIOPort  Port=3  Side=Right
  Vm : PMIOPort  Port=4  Side=Left
  connections:
  ERef R7/LConn1 -- R7/RConn1
  R2/RConn1 -- ERef R2/LConn1
  ERef R5/LConn1 -- R5/RConn1
  Op-Amp 2/RConn1 -- High-Power Op-Amp/LConn1 -- R6/LConn1
  High-Power Op-Amp/LConn2 -- M-/RConn1 -- R5/LConn1
  R2/LConn1 -- Op-Amp 1/LConn1 -- R1/RConn1
  R4/LConn1 -- Op-Amp 1/LConn2 -- R3/RConn1
  Op-Amp 2/LConn1 -- Op-Amp 1/RConn1 -- R4/RConn1
  R7/LConn1 -- Op-Amp 2/LConn2 -- R6/RConn1
  Vref/RConn1 -- R1/LConn1
  M+/RConn1 -- High-Power Op-Amp/RConn1
  Vm/RConn1 -- R3/LConn1

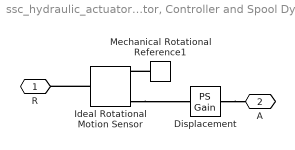
== system ssc_hydraulic_actuator_analog_control/Spool Valve/Torque Motor, Controller and Spool Dynamics/Rotation ==
  Displacement : fl_lib/Physical Signals/Functions/PS Gain  gain=G m/rad
      settings: SourceProductName=Foundation Library
  Ideal Rotational Motion Sensor : fl_lib/Mechanical/Mechanical Sensors/Ideal Rotational Motion Sensor  wrap_angle=simscape.enum.onoff.off  offset=0 rad
      settings: SourceProductName=Foundation Library
  Mechanical Rotational Reference1 : fl_lib/Mechanical/Rotational Elements/Mechanical Rotational Reference
      settings: SourceProductName=Foundation Library
  R : PMIOPort  Side=Left
  A : PMIOPort  Port=2  Side=Right
  connections:
  Mechanical Rotational Reference1/LConn1 -- Ideal Rotational Motion Sensor/RConn1
  Ideal Rotational Motion Sensor/RConn3 -- Displacement/LConn1
  Displacement/RConn1 -- A/RConn1
  Ideal Rotational Motion Sensor/LConn1 -- R/RConn1
